simulink model "gm_sampleModel2052_3_sub_sub"  (R2023a)
settings: Solver=VariableStepAuto  StartTime=0.0  StopTime=10.0  RelTol=1e-3
libraries: simulink x6, hdlsllib x6
settings Model: Creator=user1  LastModifiedBy=user1
settings OptimizationCC: BlockReduction=off  ConditionallyExecuteInputs=off
settings DebuggingCC: InheritedTsInSrcMsg=none

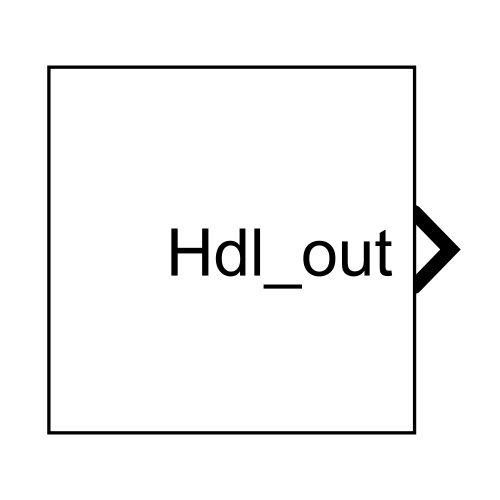
[thumbnail: Simulink's stored preview of the top-level diagram]
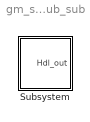
== system gm_sampleModel2052_3_sub_sub ==
  Subsystem : Subsystem

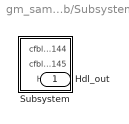
== system gm_sampleModel2052_3_sub_sub/Subsystem ==
  Subsystem : Subsystem
  Hdl_out : Outport  OutDataTypeStr=uint8

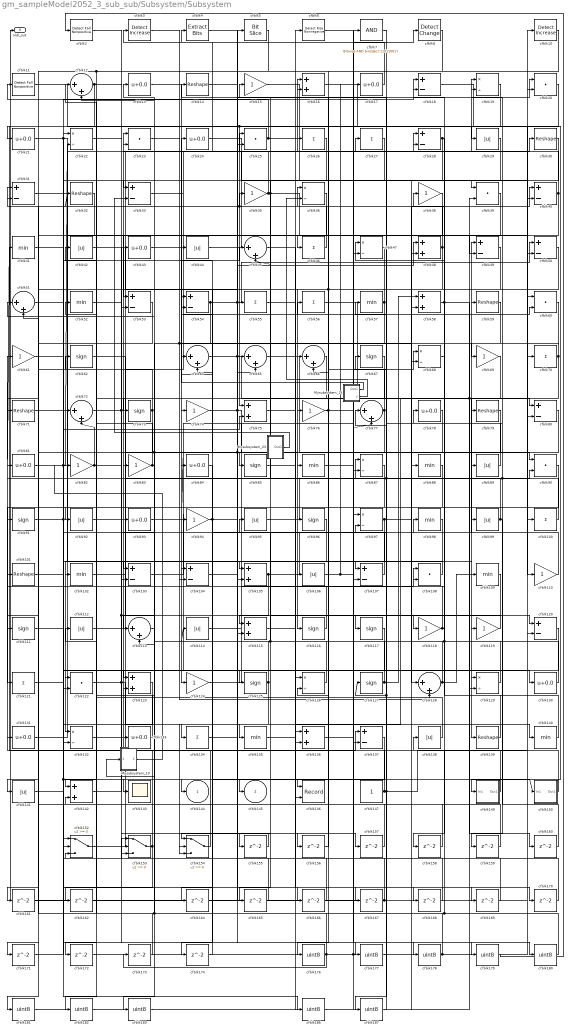
== system gm_sampleModel2052_3_sub_sub/Subsystem/Subsystem ==
  Mysubsystem_10 : Subsystem  TreatAsAtomicUnit=on  RTWFcnName=Mysubsystem_10
      settings: RTWFcnNameOpts=User specified  RTWFileNameOpts=Use function name
  Mysubsystem_15 : Subsystem  TreatAsAtomicUnit=on  RTWFcnName=Mysubsystem_15
      settings: RTWFcnNameOpts=User specified  RTWFileNameOpts=Use function name
  Mysubsystem_23 : Subsystem  TreatAsAtomicUnit=on  RTWFcnName=Mysubsystem_23
      settings: RTWFcnNameOpts=User specified  RTWFileNameOpts=Use function name
  cfblk10 : simulink/Logic and Bit Operations/Detect Increase  vinit=0.0  OutDataTypeStr=uint8
      settings: LibrarySourceBlock=|
      | hdlsllib/Logic and Bit
      | Operations/Detect
      | Increase
  cfblk{26..27,46,55..56,70,100,121,134} (9 alike) : Sum  Inputs=+  OutDataTypeStr=uint8
  cfblk{14,30,32,59,71,79,101,139} (8 alike) : Reshape
  cfblk{41,52,57,86,88,98,102,109,135,140} (10 alike) : MinMax  OutDataTypeStr=uint8
  cfblk{18,28,31,33,40,49..50,53..54,80,103..104,107,120,137} (15 alike) : Sum  Inputs=+-  OutDataTypeStr=uint8
  cfblk{16,48,58,75,105,115,123,136,142} (9 alike) : Sum  OutDataTypeStr=uint8
  cfblk{29,42,44,89,92,95,99,106,112,114,138,141} (12 alike) : Abs  OutDataTypeStr=uint8  SaturateOnIntegerOverflow=off
  cfblk{20,23,25,39,60,90,108,122} (8 alike) : DotProduct  OutDataTypeStr=uint8
  cfblk11 : hdlsllib/Logic and Bit Operations/Detect Fall Nonpositive  vinit=0  OutDataTypeStr=uint8
  cfblk{15,35,38,61,69,74,76,82..83,94,110,118..119,124} (14 alike) : Gain  OutDataTypeStr=uint8
  cfblk{62,67,73,85,91,96,111,116..117,125,127} (11 alike) : Signum
  cfblk{12,45,51,64..66,72,77,113,128} (10 alike) : Sum  Inputs=|++  OutDataTypeStr=uint8
  cfblk{19,22,36,47,68,87,97,126,129,132} (10 alike) : Product  Inputs=*/  OutDataTypeStr=uint8  RndMeth=Zero  SaturateOnIntegerOverflow=on
  cfblk{13,17,21,24,43,78,81,84,93,130..131,133} (12 alike) : Bias  Bias=0.0  SaturateOnIntegerOverflow=off
  cfblk143 : Scope
  cfblk146 : Record  FileSettingsInternal="{\"entries\":[{\"content\":{\"excelSettings\":{\"content\":{},\"type\":\"Streamout.ExcelSettings\"}},\"type\":\"Streamout.FileSettingStorage\",\"uuid\":\"\"}],\"packageUris\":[\"http:\\/\\/schema.mathworks.com\\/mf0\\/streamout_blocks\\/R2020a\"],\"version\":\"1.0\"}"  Layout=[1 1]  SignalsInternal="{\"entries\":[{\"content\":{\"signals\":[{\"content\":{\"blockPath\":[],\"dimensions\":[1],\"domain\":\"\",\"lineColor\":\"#a2142f\",\"plots\":[1],\"port\":1,\"signalID\":60473,\"signalName\":\"cfblk76\"},\"type\":\"RecordBlkView.Signal\",\"uuid\":\"\"},{\"content\":{\"blockPath\":[],\"dimensions\":[1],\"domain\":\"\",\"lineColor\":\"#139fff\",\"plots\":[1],\"port\":2,\"signalID\":60476,\"signalName\":\"cfblk74\"},\"type\":\"RecordBlkView.Signal\",\"uuid\":\"\"}]},\"type\":\"RecordBlkView.InputSignals\",\"uuid\":\"\"}],\"packageUris\":[\"http:\\/\\/schema.mathworks.com\\/mf0\\/streamout_blocks\\/R2020a\"],\"version\":\"1.0\"}"  VisualizationBindings="{\"xyplotplugin\":{\"info\":[{\"series\":[{\"bindingParametersList\":[{\"parameter\":\"X-Axis\",\"signalID\":60473,\"signalName\":\"cfblk76\"},{\"parameter\":\"Y-Axis\",\"signalID\":60476,\"signalName\":\"cfblk74\"}],\"seriesID\":28375}],\"subplotID\":1}]}}"  CompatibilityTag=XY  st=-1
  cfblk147 : Constant  OutDataTypeStr=uint8  SampleTime=-1
  cfblk149 : Subsystem
      settings: LibrarySourceBlock=|
      | hdlsllib/Ports &
      | Subsystems/Subsystem
  cfblk150 : Subsystem
      settings: LibrarySourceBlock=|
      | hdlsllib/Ports &
      | Subsystems/Subsystem
  cfblk152 : Switch  OutDataTypeStr=uint8  SaturateOnIntegerOverflow=off  InputSameDT=off
  cfblk153 : Switch  OutDataTypeStr=uint8  SaturateOnIntegerOverflow=off  InputSameDT=off
  cfblk154 : Switch  OutDataTypeStr=uint8  SaturateOnIntegerOverflow=off  InputSameDT=off
  cfblk{155..162,164..174} (19 alike) : Delay  SampleTime=1
  cfblk{176..183,186..187} (10 alike) : DataTypeConversion  OutDataTypeStr=uint8  SaturateOnIntegerOverflow=off  RndMeth=Floor
  cfblk2 : hdlsllib/Logic and Bit Operations/Detect Fall Nonpositive  vinit=0  OutDataTypeStr=uint8
  cfblk3 : simulink/Logic and Bit Operations/Detect Increase  vinit=0.0  OutDataTypeStr=uint8
      settings: LibrarySourceBlock=|
      | hdlsllib/Logic and Bit
      | Operations/Detect
      | Increase
  cfblk4 : simulink/Logic and Bit Operations/Extract Bits  bitsToExtract=Upper half  numBits=8  bitIdxRange=[0 7]  outScalingMode=Preserve fixed-point scaling
      settings: LibrarySourceBlock=|
      | hdlsllib/Logic and Bit
      | Operations/Extract Bits
  cfblk5 : hdlsllib/Logic and Bit Operations/Bit Slice  lidx=7  ridx=0
  cfblk6 : hdlsllib/Logic and Bit Operations/Detect Rise Nonnegative  vinit=0  OutDataTypeStr=uint8
  cfblk7 : simulink/Logic and Bit Operations/Bitwise Operator  logicop=AND  UseBitMask=on  BitMask=bin2dec('11011001')  BitMaskRealWorld=Stored Integer
      settings: LibrarySourceBlock=|
      | hdlsllib/Logic and Bit
      | Operations/Bitwise
      | Operator
  cfblk8 : simulink/Logic and Bit Operations/Detect Change  vinit=0  OutDataTypeStr=uint8
      settings: LibrarySourceBlock=|
      | hdlsllib/Logic and Bit
      | Operations/Detect
      | Change
  cfblk144 : Outport  OutDataTypeStr=uint8  VectorParamsAs1DForOutWhenUnconnected=off
  cfblk145 : Outport  Port=2  OutDataTypeStr=uint8  VectorParamsAs1DForOutWhenUnconnected=off
  Hdl_out : Outport  Port=3  OutDataTypeStr=uint8
  wires:
  cfblk131/1 -> cfblk30/1
  cfblk127/1 -> cfblk54/1, cfblk58/1
  cfblk69/1 -> cfblk135/1
  cfblk119/1 -> cfblk117/1
  cfblk12/1 -> cfblk104/1, cfblk137/1
  cfblk100/1 -> cfblk79/1, cfblk57/1, cfblk41/1
  cfblk47/1 -> cfblk116/1
  cfblk94/1 -> cfblk177/1, cfblk54/2
  cfblk21/1 -> cfblk129/2, cfblk46/1
  cfblk18/1 -> cfblk149/1(In1)
  cfblk128/1 -> cfblk109/1, cfblk77/1
  cfblk56/1 -> cfblk139/1
  cfblk52/1 -> cfblk168/1, cfblk115/2
  cfblk40/1 -> cfblk153/3, cfblk23/1
  cfblk154/1 -> cfblk23/2
  cfblk13/1 -> cfblk124/1
  cfblk20/1 -> cfblk91/1, cfblk75/1
  cfblk81/1 -> cfblk104/2, cfblk22/2
  cfblk62/1 -> cfblk86/1
  cfblk25/1 -> cfblk70/1, cfblk11/1
  cfblk95/1 -> cfblk49/1
  cfblk114/1 -> cfblk8/1
  cfblk30/1 -> cfblk58/2
  cfblk152/1 -> cfblk25/1
  cfblk84/1 -> cfblk134/1
  cfblk96/1 -> cfblk132/1
  cfblk43/1 -> cfblk74/1
  cfblk153/1 -> cfblk172/1, cfblk61/1
  cfblk110/1 -> cfblk89/1
  cfblk53/1 -> cfblk71/1
  cfblk98/1 -> cfblk102/1
  cfblk64/1 -> cfblk27/1, cfblk80/1
  cfblk112/1 -> cfblk56/1
  cfblk72/1 -> cfblk129/1, cfblk118/1
  cfblk140/1 -> cfblk47/1
  cfblk46/1 -> cfblk36/1
  cfblk92/1 -> cfblk5/1
  cfblk129/1 -> cfblk12/2, cfblk108/1
  cfblk113/1 -> cfblk13/1
  cfblk150/1(Out1) -> cfblk112/1
  cfblk115/1 -> cfblk28/1
  cfblk68/1 -> cfblk38/1
  cfblk44/1 -> cfblk16/1
  cfblk17/1 -> cfblk3/1
  cfblk31/1 -> cfblk119/1
  cfblk10/1 -> cfblk176/1
  cfblk116/1 -> cfblk83/1
  cfblk138/1 -> cfblk62/1
  cfblk11/1 -> cfblk100/1
  cfblk5/1 -> cfblk141/1, cfblk122/1
  cfblk27/1 -> cfblk85/1
  cfblk7/1 -> cfblk187/1
  cfblk24/1 -> cfblk39/1
  cfblk15/1 -> cfblk128/1
  cfblk108/1 -> cfblk105/1
  cfblk126/1 -> cfblk51/1
  cfblk99/1 -> cfblk159/1, cfblk15/1
  cfblk73/1 -> cfblk31/2, cfblk142/1
  cfblk120/1 -> cfblk122/2
  cfblk89/1 -> cfblk14/1
  cfblk147/1 -> cfblk66/2, cfblk20/2, cfblk87/1
  cfblk118/1 -> cfblk78/1, cfblk44/1
  cfblk103/1 -> cfblk68/1
  cfblk33/1 -> cfblk19/1
  cfblk4/1 -> cfblk49/2
  cfblk87/1 -> cfblk121/1
  cfblk124/1 -> cfblk108/2
  cfblk39/1 -> cfblk53/1
  cfblk136/1 -> cfblk97/1
  cfblk93/1 -> cfblk130/1
  cfblk28/1 -> cfblk158/1, cfblk132/2
  cfblk149/1(Out1) -> cfblk81/1
  cfblk55/1 -> cfblk96/1
  cfblk23/1 -> cfblk128/2
  cfblk82/1 -> cfblk107/2, cfblk72/2
  cfblk106/1 -> cfblk17/1, cfblk47/2
  cfblk86/1 -> cfblk60/2
  cfblk77/1 -> cfblk26/1, cfblk111/1
  cfblk58/1 -> cfblk28/2, cfblk160/1, cfblk80/2
  cfblk139/1 -> cfblk18/1
  cfblk48/1 -> cfblk84/1, cfblk32/1, cfblk35/1
  cfblk26/1 -> cfblk65/1
  cfblk35/1 -> cfblk4/1, cfblk110/1, cfblk45/2
  cfblk105/1 -> cfblk115/1, cfblk99/1
  cfblk83/1 -> cfblk31/1, Mysubsystem_10/1(In1)
  cfblk76/1 -> cfblk140/1, cfblk146/1
  cfblk78/1 -> cfblk103/2, cfblk113/1
  cfblk111/1 -> cfblk144/1
  cfblk67/1 -> cfblk87/2, cfblk92/1
  cfblk42/1 -> cfblk65/2
  cfblk22/1 -> cfblk133/1
  cfblk54/1 -> cfblk103/1, cfblk48/1, cfblk50/1
  cfblk97/1 -> cfblk40/1, cfblk125/1
  cfblk102/1 -> cfblk50/2
  cfblk65/1 -> cfblk90/1
  cfblk66/1 -> cfblk145/1
  cfblk80/1 -> cfblk113/2
  cfblk79/1 -> cfblk94/1, cfblk105/2
  cfblk60/1 -> cfblk73/1
  cfblk130/1 -> cfblk114/1, cfblk95/1
  cfblk91/1 -> cfblk18/2, cfblk170/1, cfblk150/1(In1)
  cfblk19/1 -> cfblk21/1
  cfblk57/1 -> cfblk136/2, cfblk55/1
  cfblk16/1 -> cfblk29/1
  cfblk134/1 -> cfblk20/1
  cfblk29/1 -> cfblk33/1
  cfblk101/1 -> cfblk45/1
  cfblk45/1 -> cfblk66/1
  cfblk70/1 -> cfblk69/1, cfblk106/1
  cfblk49/1 -> cfblk165/1, cfblk76/1
  cfblk142/1 -> cfblk43/1
  cfblk135/1 -> cfblk90/2
  cfblk71/1 -> cfblk143/1
  cfblk3/1 -> cfblk120/1, cfblk68/2
  cfblk2/1 -> cfblk178/1
  cfblk85/1 -> cfblk137/2
  cfblk123/1 -> cfblk152/2
  cfblk125/1 -> cfblk101/1, cfblk154/2
  cfblk121/1 -> cfblk98/1
  cfblk6/1 -> cfblk180/1
  cfblk59/1 -> cfblk107/1
  cfblk8/1 -> cfblk53/2
  cfblk133/1 -> cfblk52/1
  cfblk74/1 -> cfblk146/2, cfblk59/1, cfblk126/1
  cfblk51/1 -> cfblk123/1
  cfblk141/1 -> cfblk75/2
  cfblk107/1 -> cfblk64/2
  cfblk122/1 -> cfblk156/1, cfblk154/3
  cfblk109/1 -> cfblk155/1
  cfblk155/1 -> cfblk154/1
  cfblk156/1 -> cfblk126/2
  cfblk132/1 -> cfblk157/1
  cfblk157/1 -> cfblk16/2
  cfblk158/1 -> cfblk51/2
  cfblk159/1 -> cfblk97/2
  cfblk160/1 -> cfblk19/2
  cfblk50/1 -> cfblk161/1
  cfblk161/1 -> cfblk60/1
  cfblk38/1 -> cfblk162/1
  cfblk162/1 -> cfblk142/2
  cfblk117/1 -> cfblk164/1
  cfblk164/1 -> cfblk25/2
  cfblk165/1 -> cfblk153/2
  cfblk14/1 -> cfblk166/1
  cfblk166/1 -> cfblk136/1
  cfblk75/1 -> cfblk167/1
  cfblk167/1 -> Hdl_out/1, cfblk153/1
  cfblk168/1 -> cfblk22/1
  cfblk104/1 -> cfblk169/1
  cfblk169/1 -> cfblk152/1
  cfblk170/1 -> cfblk123/2
  cfblk32/1 -> cfblk171/1
  cfblk171/1 -> cfblk72/1
  cfblk172/1 -> cfblk40/2
  cfblk173/1 -> cfblk152/3
  cfblk137/1 -> cfblk174/1
  cfblk174/1 -> cfblk64/1
  cfblk176/1 -> cfblk131/1, cfblk173/1, cfblk77/2, cfblk48/2
  cfblk177/1 -> cfblk10/1
  cfblk178/1 -> cfblk42/1, cfblk120/2
  cfblk41/1 -> cfblk179/1
  cfblk179/1 -> cfblk2/1
  cfblk180/1 -> cfblk138/1, cfblk12/1, cfblk93/1
  cfblk36/1 -> cfblk181/1
  cfblk181/1 -> cfblk6/1
  cfblk88/1 -> cfblk182/1
  cfblk182/1 -> cfblk39/2
  cfblk90/1 -> cfblk183/1
  cfblk183/1 -> cfblk88/1
  cfblk61/1 -> cfblk186/1
  cfblk186/1 -> cfblk7/1
  cfblk187/1 -> cfblk127/1, cfblk67/1
  Mysubsystem_10/1(Out1) -> cfblk82/1
  Mysubsystem_15/1(Out1) -> cfblk24/1
  Mysubsystem_15/2(y) -> cfblk36/2
  Mysubsystem_23/1(Out1) -> cfblk33/2

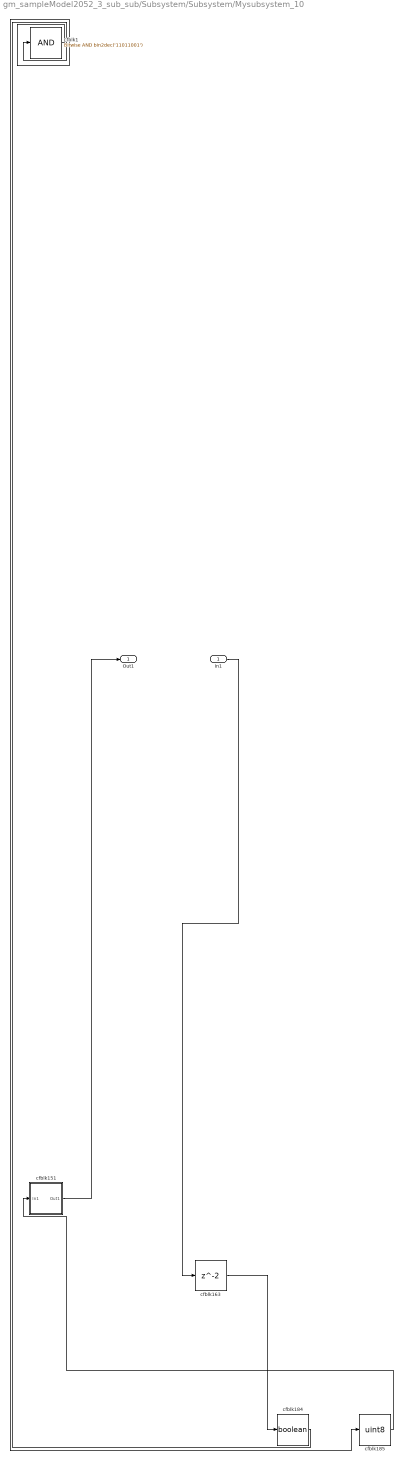
== system gm_sampleModel2052_3_sub_sub/Subsystem/Subsystem/Mysubsystem_10 ==
  In1 : Inport
  cfblk1 : simulink/Logic and Bit Operations/Bitwise Operator  logicop=AND  UseBitMask=on  BitMask=bin2dec('11011001')  BitMaskRealWorld=Stored Integer
      settings: LibrarySourceBlock=|
      | hdlsllib/Logic and Bit
      | Operations/Bitwise
      | Operator
  cfblk151 : Subsystem
      settings: LibrarySourceBlock=|
      | hdlsllib/Ports &
      | Subsystems/Subsystem
  cfblk163 : Delay  SampleTime=1
  cfblk184 : DataTypeConversion  OutDataTypeStr=boolean  SaturateOnIntegerOverflow=off  RndMeth=Floor
  cfblk185 : DataTypeConversion  OutDataTypeStr=uint8  SaturateOnIntegerOverflow=off  RndMeth=Floor
  Out1 : Outport
  wires:
  cfblk151/1(Out1) -> Out1/1
  cfblk184/1 -> cfblk1/1
  cfblk185/1 -> cfblk151/1(In1)
  cfblk163/1 -> cfblk184/1
  In1/1 -> cfblk163/1
  cfblk1/1 -> cfblk185/1

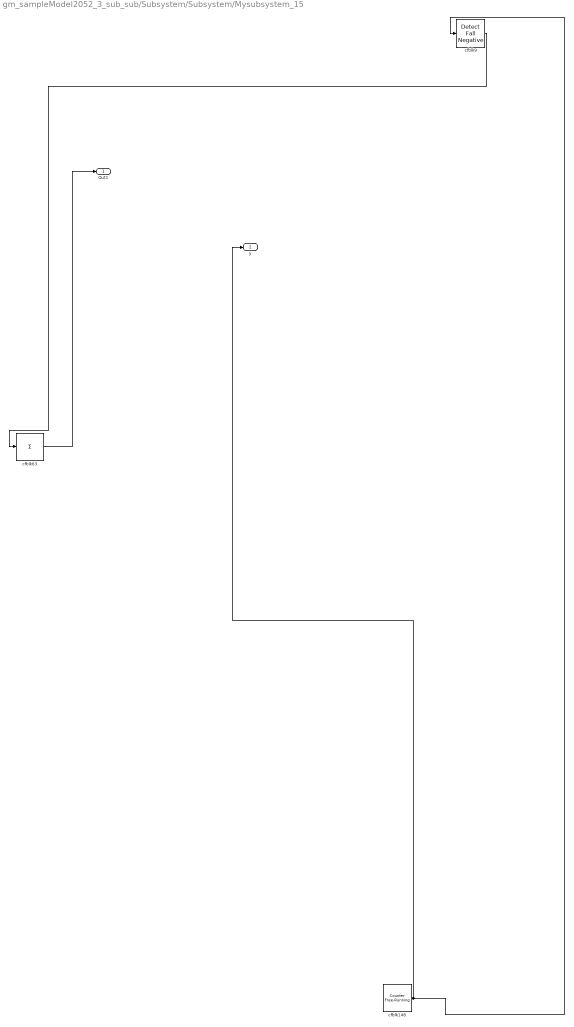
== system gm_sampleModel2052_3_sub_sub/Subsystem/Subsystem/Mysubsystem_15 ==
  cfblk148 : hdlsllib/Sources/Counter Free-Running  NumBits=16  tsamp=-1
  cfblk63 : Sum  Inputs=+
  cfblk9 : hdlsllib/Logic and Bit Operations/Detect Fall Negative  vinit=0  OutDataTypeStr=boolean
  Out1 : Outport
  y : Outport  Port=2
  wires:
  cfblk63/1 -> Out1/1
  cfblk9/1 -> cfblk63/1
  cfblk148/1 -> cfblk9/1, y/1

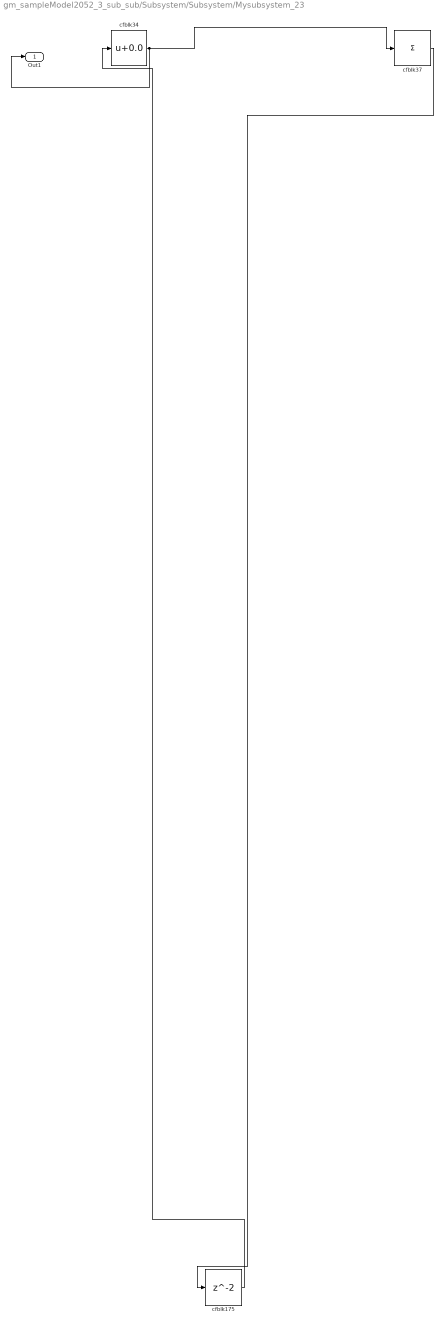
== system gm_sampleModel2052_3_sub_sub/Subsystem/Subsystem/Mysubsystem_23 ==
  cfblk175 : Delay  SampleTime=1
  cfblk34 : Bias  Bias=0.0  SaturateOnIntegerOverflow=off
  cfblk37 : Sum  Inputs=+
  Out1 : Outport
  wires:
  cfblk175/1 -> cfblk34/1
  cfblk37/1 -> cfblk175/1
  cfblk34/1 -> cfblk37/1, Out1/1

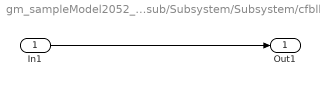
== system gm_sampleModel2052_3_sub_sub/Subsystem/Subsystem/cfblk149 ==
  In1 : Inport
  Out1 : Outport
  wires:
  In1/1 -> Out1/1

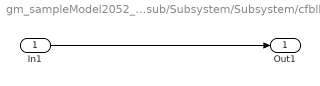
== system gm_sampleModel2052_3_sub_sub/Subsystem/Subsystem/cfblk150 ==
  In1 : Inport
  Out1 : Outport
  wires:
  In1/1 -> Out1/1

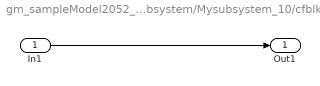
== system gm_sampleModel2052_3_sub_sub/Subsystem/Subsystem/Mysubsystem_10/cfblk151 ==
  In1 : Inport
  Out1 : Outport
  wires:
  In1/1 -> Out1/1
